simulink model "pierwsza_polowa"  (R2018b)
settings: Solver=VariableStepAuto  StartTime=0.0  StopTime=100  RelTol=1e-3
values from neighbouring files (symbols this model uses):
  tp = 1    [dane.m]
undefined symbols (not defined in the file or in its folder): k
settings Model: Creator=podstawy  LastModifiedBy=podstawy

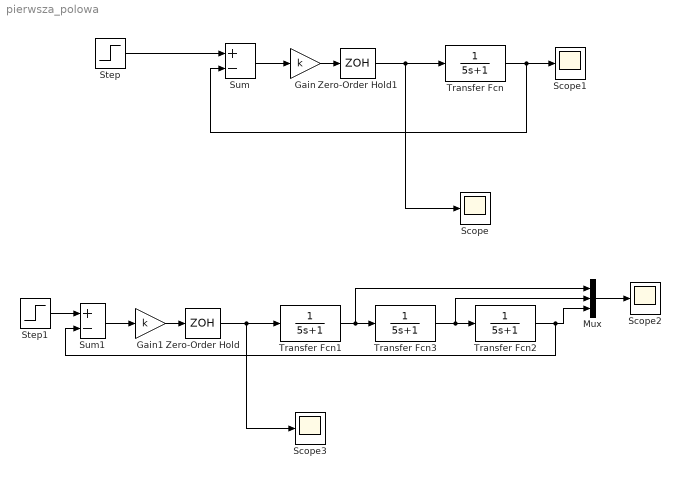
== system pierwsza_polowa ==
  Gain : Gain  Gain=k
  Gain1 : Gain  Gain=k
  Mux : Mux  Inputs=3
  Scope{,1..3} (4 alike) : Scope
  Step : Step  SampleTime=0
  Step1 : Step  SampleTime=0
  Sum : Sum  Inputs=+-
  Sum1 : Sum  Inputs=+-
  Transfer Fcn{,1..3} (4 alike) : TransferFcn  Denominator=[5 1]
  Zero-Order Hold : ZeroOrderHold  SampleTime=tp
  Zero-Order Hold1 : ZeroOrderHold  SampleTime=tp
  wires:
  Step/1 -> Sum/1
  Sum/1 -> Gain/1
  Transfer Fcn/1 -> Sum/2, Scope1/1
  Step1/1 -> Sum1/1
  Sum1/1 -> Gain1/1
  Transfer Fcn1/1 -> Mux/1, Transfer Fcn3/1
  Transfer Fcn3/1 -> Mux/2, Transfer Fcn2/1
  Mux/1 -> Scope2/1
  Transfer Fcn2/1 -> Mux/3, Sum1/2
  Gain1/1 -> Zero-Order Hold/1
  Zero-Order Hold/1 -> Scope3/1, Transfer Fcn1/1
  Gain/1 -> Zero-Order Hold1/1
  Zero-Order Hold1/1 -> Scope/1, Transfer Fcn/1
